simulink model "d_kundur2"  (Simulink 5.1)
settings: Solver=ode45  StartTime=0.0  StopTime=10.0  RelTol=1e-3
libraries: fm_lib x20
settings Model: Creator=fmilano  LastModifiedBy=fmilano  ExtModeAutoUpdateStatusClock=off  SignalLoggingName=logsout  BooleanDataType=on  RTWOptions="-aEnforceIntegerDowncast=1 -aFoldNonRolledExpr=1 -aInlineInvariantSignals=1 -aInlineParameters=0 -aLocalBlockOutputs=1 -aRollThreshold=5 -aZeroInternalMemoryAtStartup=1 -aZeroExternalMemoryAtStartup=1 -aInitFltsAndDblsToZero=1 -aForceBlockIOInitOptimize=0 -aGenerateReport=0 -aGenCodeOnly=0 -aRTWVerbose=1 -aIncludeHyperlinkInReport=0 -aLaunchReport=0 -aGenerateTraceInfo=0  -aForceParamTrailComments=0 -aGenerateComments=1 -aIgnoreCustomStorageClasses=1 -aIncHierarchyInIds=0 -aMaxRTWIdLen=31 -aShowEliminatedStatements=0 -aIncDataTypeInIds=0 -aInsertBlockDesc=0 -aIgnoreTestpoints=0 -aSimulinkBlockComments=1 -aInlinedPrmAccess=\"Literals\"  -aSuppressErrorStatus=0 -aModelReferenceCompliant=1 -aParenthesesLevel=\"Nominal\" -aModelStepFunctionPrototypeControlCompliant=0 -aPortableWordSizes=0 -aParMdlRefBuildCompliant=1 -aSupportNonInlinedSFcns=1 -aSupportContinuousTime=1 -aSupportComplex=1 -aSupportNonFinite=1 -aSupportAbsoluteTime=1 -aMultiwordLength=2048 -aTargetPreCompLibLocation=\"\" -aTargetLibSuffix=\"\" -aTargetFunctionLibrary=\"ANSI_C\" -aTargetFcnLib=\"ansi_tfl_tmw.mat\" -aMultiInstanceERTCode=0 -aLogVarNameModifier=\"rt_\" -aERTFirstTimeCompliant=0 -aIsPILTarget=0 -aCombineOutputUpdateFcns=0 -aGenerateASAP2=0 -aGenerateClassInterface=0 -aGenerateTestInterfaces=0 -aGenerateSampleERTMain=0 -aGenerateFullHeader=1 -aUtilityFuncGeneration=\"Auto\" -aIncludeFileDelimiter=\"Auto\" -aIncludeMdlTerminateFcn=1 -aPurelyIntegerCode=0 -aAutosarCompliant=0 -aERTCustomFileBanners=0 -aRTWCAPIStates=0 -aRTWCAPIParams=0 -aRTWCAPISignals=0 -aMatFileLogging=1 -aCompOptLevelCompliant=0 -aCPPClassGenCompliant=0 -aExtModeIntrfLevel=\"Level1\" -aExtModeMexFile=\"ext_comm\" -aExtModeTransport=0 -aExtModeStaticAllocSize=1000000 -aExtModeTesting=0 -aExtModeStaticAlloc=0 -aExtMode=0 -aERTMultiwordLength=256 -aERTMultiwordTypeDef=\"System defined\"  -aGenerateTraceInfo=0 -aGenerateTraceInfo=0 -aGenerateTraceInfo=0 -aGenerateTraceInfo=0"

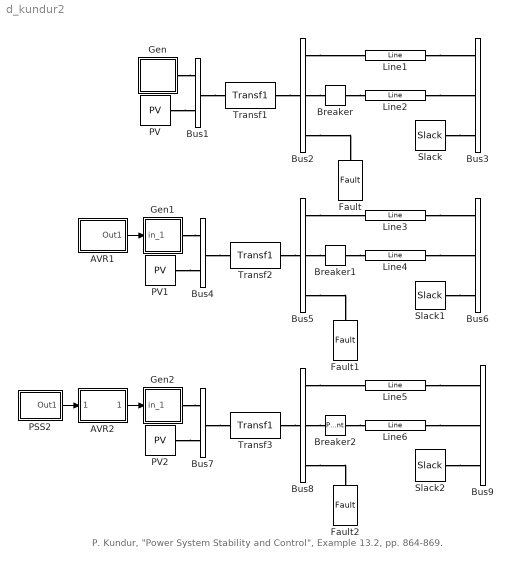
== system d_kundur2 ==
  note: P. Kundur, "Power System Stability and Control", Example 13.2, pp. 864-869.
  AVR1 : Subsystem  Tag=PSATblock  Description=Controls  mask(Exc){p2q=3, p3q=7.00, p4q=-6.40, p5q=200, p6q=1, p7q=1, p8q=1.00, p9q=0, p10q=0.0001, p11q=0.015, p12_13q=[0.0006  0.9], in=0}
      mask prompts: p2q "Automatic Voltage Regulator Type"; p3q "Maximum Regulator Voltage [p.u.]"; p4q "Minimum Regulator Voltage [p.u.]"; p5q "Regulator Gain [p.u./p.u.]"; p6q "Regulator Pole T2 [s]"; p7q "Regulator Zero T1 [s]"; p8q "Second Regulator Pole T3 [s]"; p9q "Allow signal V/V0 [0 for disabling signal]"; p10q "Time Constant of the Field Circuit Td [s]"; p11q "Time Delay of the Measurement System Tr [s]"; p12_13q "Coefficient of the Ceiling Function (A B)"; in "Number of input signals"
      mask help: This block defines an Automatic Voltage Regulator.
      mask init:
      | fm_inout
      | [x,y] = fm_draw('R');
      mask Help:
      | This block defines an Automatic Voltage Regulator.
      | There are three kind of regulators:
      | 
      | Type 1:
      | 
      |      IEEE Model 1
      | 
      | Type 2:
      | 
      |      IEEE Model 2
      | 
      | Type 3:
      | 
      |      IEEE Model 3
      mask StyleString: popup(1|2|3),edit,edit,edit,edit,edit,edit,edit,edit,edit,edit,popup(0|1|2|3)
      mask CallbackString: fm_block|||||||||||
      mask Display:
      | plot([-1.8 4.1 4.1 -1.8 -1.8],[-1.5 -1.5 1.5 1.5 -1.5])
      | color('red')
      | plot([-1.3 -0.5],[-1 1],[-0.5 0.3],[1 -1],[-0.9 -0.1],[0.0 0.0])
      | plot(2.8+1.3*x,2*y,1.5+[-1.3 -0.5],[1 -1],1.5+[-0.5 0.3],[-1 1])
  AVR2 : Subsystem  Tag=PSATblock  Description=Controls  mask(Exc){p2q=3, p3q=7.00, p4q=-6.40, p5q=200, p6q=1, p7q=1, p8q=1.00, p9q=0, p10q=0.0001, p11q=0.015, p12_13q=[0.0006  0.9], in=1}
      mask prompts: p2q "Automatic Voltage Regulator Type"; p3q "Maximum Regulator Voltage [p.u.]"; p4q "Minimum Regulator Voltage [p.u.]"; p5q "Regulator Gain [p.u./p.u.]"; p6q "Regulator Pole T2 [s]"; p7q "Regulator Zero T1 [s]"; p8q "Second Regulator Pole T3 [s]"; p9q "Allow signal V/V0 [0 for disabling signal]"; p10q "Time Constant of the Field Circuit Td [s]"; p11q "Time Delay of the Measurement System Tr [s]"; p12_13q "Coefficient of the Ceiling Function (A B)"; in "Number of input signals"
      mask help: This block defines an Automatic Voltage Regulator.
      mask init:
      | fm_inout
      | [x,y] = fm_draw('R');
      mask Help:
      | This block defines an Automatic Voltage Regulator.
      | There are three kind of regulators:
      | 
      | Type 1:
      | 
      |      IEEE Model 1
      | 
      | Type 2:
      | 
      |      IEEE Model 2
      | 
      | Type 3:
      | 
      |      IEEE Model 3
      mask StyleString: popup(1|2|3),edit,edit,edit,edit,edit,edit,edit,edit,edit,edit,popup(0|1|2|3)
      mask CallbackString: fm_block|||||||||||
      mask Display:
      | plot([-1.8 4.1 4.1 -1.8 -1.8],[-1.5 -1.5 1.5 1.5 -1.5])
      | color('red')
      | plot([-1.3 -0.5],[-1 1],[-0.5 0.3],[1 -1],[-0.9 -0.1],[0.0 0.0])
      | plot(2.8+1.3*x,2*y,1.5+[-1.3 -0.5],[1 -1],1.5+[-0.5 0.3],[-1 1])
  Breaker : fm_lib/Faults &  Breakers/Breaker  Tag=PSATblock  Description=Faults & Breakers  PhysicalDomain=psatdomain  SubClassName=unknown  LeftPortType=p1  RightPortType=p1  LConnTagsString=__newl0  RConnTagsString=__newr0  p3_4_5q="[2220  400  60]"  p6q=on  p7q=0.57  p8q=100  p9q=on  p10q=on
  Breaker1 : fm_lib/Faults &  Breakers/Breaker  Tag=PSATblock  Description=Faults & Breakers  PhysicalDomain=psatdomain  SubClassName=unknown  LeftPortType=p1  RightPortType=p1  LConnTagsString=__newl0  RConnTagsString=__newr0  p3_4_5q="[2220  400  60]"  p6q=on  p7q=0.57  p8q=100  p9q=on  p10q=on
  Breaker2 : PMComponent  Tag=PSATblock  Description=Faults & Breakers  PhysicalDomain=psatdomain  LeftPortType=p1  RightPortType=p1  LConnTagsString=__newl0  RConnTagsString=__newr0  mask(Breaker){p3_4_5q=[2220  400  60], p6q=on, p7q=0.57, p8q=100}
      mask prompts: p3_4_5q "Power, Voltage and Frequency Ratings [MVA, kV, Hz]"; p6q "Initially close"; p7q "First intervention time [s]"; p8q "Second intervention time [s]"
      mask help: This block defines a breaker.
      mask CallbackString: |fm_block||
      mask Display: plot([1 2 2 1 1],[-1 -1 1 1 -1]),color('red'),plot([1 2],[-1 1],[2 1],[-1 1])
  Bus1 : PMComponent  Tag=PSATblock  Description=Connection  PhysicalDomain=psatdomain  LeftPortType=p1  RightPortType=p1  LConnTagsString=__newl0|__newl1  RConnTagsString=__newr0  mask(Bus){in=2, out=1, p2q=400, p3_4q=[1.00   0.00], p5q=1, p6q=1}
      mask prompts: in "Number of inputs:"; out "Number of outputs:"; p2q "Voltage Rating [kV]"; p3_4q "Voltage initial guess [p.u.  rad]"; p5q "Area number"; p6q "Region number"
      mask help: Bus block.
      mask init:
      | fm_inout
      mask CallbackString: ||||fm_block|
      mask Display: plot([0 1 1 0 0],[0 0 1 1 0])
  Bus2 : PMComponent  Tag=PSATblock  Description=Connection  PhysicalDomain=psatdomain  LeftPortType=p1  RightPortType=p1  LConnTagsString=__newl0  RConnTagsString=__newr0|__newr1|__newr2  mask(Bus){in=1, out=3, p2q=400, p3_4q=[1.00   0.00], p5q=1, p6q=1}
      mask prompts: in "Number of inputs:"; out "Number of outputs:"; p2q "Voltage Rating [kV]"; p3_4q "Voltage initial guess [p.u.  rad]"; p5q "Area number"; p6q "Region number"
      mask help: Bus block.
      mask init:
      | fm_inout
      mask CallbackString: ||||fm_block|
      mask Display: plot([0 1 1 0 0],[0 0 1 1 0])
  Bus3 : PMComponent  Tag=PSATblock  Description=Connection  PhysicalDomain=psatdomain  LeftPortType=p1  RightPortType=p1  LConnTagsString=__newl0|__newl1|__newl2  mask(Bus){in=3, out=0, p2q=400, p3_4q=[1.00   0.00], p5q=1, p6q=1}
      mask prompts: in "Number of inputs:"; out "Number of outputs:"; p2q "Voltage Rating [kV]"; p3_4q "Voltage initial guess [p.u.  rad]"; p5q "Area number"; p6q "Region number"
      mask help: Bus block.
      mask init:
      | fm_inout
      mask CallbackString: ||||fm_block|
      mask Display: plot([0 1 1 0 0],[0 0 1 1 0])
  Bus4 : PMComponent  Tag=PSATblock  Description=Connection  PhysicalDomain=psatdomain  LeftPortType=p1  RightPortType=p1  LConnTagsString=__newl0|__newl1  RConnTagsString=__newr0  mask(Bus){in=2, out=1, p2q=400, p3_4q=[1.00   0.00], p5q=1, p6q=1}
      mask prompts: in "Number of inputs:"; out "Number of outputs:"; p2q "Voltage Rating [kV]"; p3_4q "Voltage initial guess [p.u.  rad]"; p5q "Area number"; p6q "Region number"
      mask help: Bus block.
      mask init:
      | fm_inout
      mask CallbackString: ||||fm_block|
      mask Display: plot([0 1 1 0 0],[0 0 1 1 0])
  Bus5 : PMComponent  Tag=PSATblock  Description=Connection  PhysicalDomain=psatdomain  LeftPortType=p1  RightPortType=p1  LConnTagsString=__newl0  RConnTagsString=__newr0|__newr1|__newr2  mask(Bus){in=1, out=3, p2q=400, p3_4q=[1.00   0.00], p5q=1, p6q=1}
      mask prompts: in "Number of inputs:"; out "Number of outputs:"; p2q "Voltage Rating [kV]"; p3_4q "Voltage initial guess [p.u.  rad]"; p5q "Area number"; p6q "Region number"
      mask help: Bus block.
      mask init:
      | fm_inout
      mask CallbackString: ||||fm_block|
      mask Display: plot([0 1 1 0 0],[0 0 1 1 0])
  Bus6 : PMComponent  Tag=PSATblock  Description=Connection  PhysicalDomain=psatdomain  LeftPortType=p1  RightPortType=p1  LConnTagsString=__newl0|__newl1|__newl2  mask(Bus){in=3, out=0, p2q=400, p3_4q=[1.00   0.00], p5q=1, p6q=1}
      mask prompts: in "Number of inputs:"; out "Number of outputs:"; p2q "Voltage Rating [kV]"; p3_4q "Voltage initial guess [p.u.  rad]"; p5q "Area number"; p6q "Region number"
      mask help: Bus block.
      mask init:
      | fm_inout
      mask CallbackString: ||||fm_block|
      mask Display: plot([0 1 1 0 0],[0 0 1 1 0])
  Bus7 : PMComponent  Tag=PSATblock  Description=Connection  PhysicalDomain=psatdomain  LeftPortType=p1  RightPortType=p1  LConnTagsString=__newl0|__newl1  RConnTagsString=__newr0  mask(Bus){in=2, out=1, p2q=400, p3_4q=[1.00   0.00], p5q=1, p6q=1}
      mask prompts: in "Number of inputs:"; out "Number of outputs:"; p2q "Voltage Rating [kV]"; p3_4q "Voltage initial guess [p.u.  rad]"; p5q "Area number"; p6q "Region number"
      mask help: Bus block.
      mask init:
      | fm_inout
      mask CallbackString: ||||fm_block|
      mask Display: plot([0 1 1 0 0],[0 0 1 1 0])
  Bus8 : PMComponent  Tag=PSATblock  Description=Connection  PhysicalDomain=psatdomain  LeftPortType=p1  RightPortType=p1  LConnTagsString=__newl0  RConnTagsString=__newr0|__newr1|__newr2  mask(Bus){in=1, out=3, p2q=400, p3_4q=[1.00   0.00], p5q=1, p6q=1}
      mask prompts: in "Number of inputs:"; out "Number of outputs:"; p2q "Voltage Rating [kV]"; p3_4q "Voltage initial guess [p.u.  rad]"; p5q "Area number"; p6q "Region number"
      mask help: Bus block.
      mask init:
      | fm_inout
      mask CallbackString: ||||fm_block|
      mask Display: plot([0 1 1 0 0],[0 0 1 1 0])
  Bus9 : PMComponent  Tag=PSATblock  Description=Connection  PhysicalDomain=psatdomain  LeftPortType=p1  RightPortType=p1  LConnTagsString=__newl0|__newl1|__newl2  mask(Bus){in=3, out=0, p2q=400, p3_4q=[1.00   0.00], p5q=1, p6q=1}
      mask prompts: in "Number of inputs:"; out "Number of outputs:"; p2q "Voltage Rating [kV]"; p3_4q "Voltage initial guess [p.u.  rad]"; p5q "Area number"; p6q "Region number"
      mask help: Bus block.
      mask init:
      | fm_inout
      mask CallbackString: ||||fm_block|
      mask Display: plot([0 1 1 0 0],[0 0 1 1 0])
  Fault : fm_lib/Faults &  Breakers/Fault  Tag=PSATblock  Description=Faults & Breakers  Orientation=down  PhysicalDomain=psatdomain  SubClassName=unknown  LeftPortType=p1  RightPortType=p1  LConnTagsString=__newl0  p2_3_4q="[2220  400  60]"  p5q=0.5  p6q=0.57  p7q=0  p8q=1e-5
  Fault1 : fm_lib/Faults &  Breakers/Fault  Tag=PSATblock  Description=Faults & Breakers  Orientation=down  PhysicalDomain=psatdomain  SubClassName=unknown  LeftPortType=p1  RightPortType=p1  LConnTagsString=__newl0  p2_3_4q="[2220  400  60]"  p5q=0.5  p6q=0.57  p7q=0  p8q=1e-5
  Fault2 : fm_lib/Faults &  Breakers/Fault  Tag=PSATblock  Description=Faults & Breakers  Orientation=down  PhysicalDomain=psatdomain  SubClassName=unknown  LeftPortType=p1  RightPortType=p1  LConnTagsString=__newl0  p2_3_4q="[2220  400  60]"  p5q=0.5  p6q=0.57  p7q=0  p8q=1e-5
  Gen : Subsystem  Tag=PSATblock  Description=Machines  mask(Syn){p2_3_4q=[2220  400   60], p5q=6, p7_6q=[0.003  0.15], p8_9_10q=[1.81  0.30  0.23], p11_12q=[8.00  0.03], p13_14_15q=[1.76  0.65  0.25], p16_17q=[1.00  0.07], p18_19q=[7.00  0.00], p20_21q=[0.00  0.00], p22_23q=[1.00  1.00], p24q=0.00, p25_26q=[0.05 0.1], in=0, p27q=0, p28q=on}
      mask prompts: p2_3_4q "Power, voltage and frequency ratings [MVA, kV, Hz]"; p5q "Machine Dynamic Order"; p7_6q "resistance ra and leakage reactance xl [p.u. p.u.]"; p8_9_10q "d-axis reactances Xd, X'd X"d [p.u.,p.u.,p.u.]"; p11_12q "d-axis open circuit time constants T'd0 and T"d0 [s, s]"; p13_14_15q "q-axis reactances Xq, X'q, X"q [p.u.  p.u.  p.u.]"; p16_17q "q-axis open circuit time constants T'q0 and T"q0 [s s]"; p18_19q "Inertia (M = 2H) and Damping [s, p.u.]"; p20_21q "Speed and active power additional signals Kw and Kp [p.u., p.u.]"; p22_23q "Percentage of active and reactive powers at bus [p.u. p.u.]"; p24q "d-axis additional circuit leakage time constant Taa [s]"; p25_26q "Saturation coefficients S(1.0) and S(1.2)"; in "Number of input signals"; p27q "COI number"; p28q "Connected"
      mask help: This block defines a fourth order synchronous machine.
      mask init:
      | fm_inout
      | [x,y] = fm_draw('circle');
      | [xg,yg] = fm_draw('G');
      | [xs,ys] = fm_draw('sinus');
      mask StyleString: edit,popup(8|6|5.3|5.2|5.1|4|3|2),edit,edit,edit,edit,edit,edit,edit,edit,edit,edit,popup(0|1|2),edit,checkbox
      mask CallbackString: |fm_block|||||||||||||fm_block
      mask Display:
      | plot(x+1.4,y,0.12*xs+1,0.15*ys-0.6)
      | color('blue')
      | plot(1.4+0.45*xg,0.3+0.45*yg)
  Gen1 : Subsystem  Tag=PSATblock  Description=Machines  mask(Syn){p2_3_4q=[2220  400   60], p5q=6, p7_6q=[0.003  0.15], p8_9_10q=[1.81  0.30  0.23], p11_12q=[8.00  0.03], p13_14_15q=[1.76  0.65  0.25], p16_17q=[1.00  0.07], p18_19q=[7.00  0.00], p20_21q=[0.00  0.00], p22_23q=[1.00  1.00], p24q=0.00, p25_26q=[0.05 0.1], in=1, p27q=0, p28q=on}
      mask prompts: p2_3_4q "Power, voltage and frequency ratings [MVA, kV, Hz]"; p5q "Machine Dynamic Order"; p7_6q "resistance ra and leakage reactance xl [p.u. p.u.]"; p8_9_10q "d-axis reactances Xd, X'd X"d [p.u.,p.u.,p.u.]"; p11_12q "d-axis open circuit time constants T'd0 and T"d0 [s, s]"; p13_14_15q "q-axis reactances Xq, X'q, X"q [p.u.  p.u.  p.u.]"; p16_17q "q-axis open circuit time constants T'q0 and T"q0 [s s]"; p18_19q "Inertia (M = 2H) and Damping [s, p.u.]"; p20_21q "Speed and active power additional signals Kw and Kp [p.u., p.u.]"; p22_23q "Percentage of active and reactive powers at bus [p.u. p.u.]"; p24q "d-axis additional circuit leakage time constant Taa [s]"; p25_26q "Saturation coefficients S(1.0) and S(1.2)"; in "Number of input signals"; p27q "COI number"; p28q "Connected"
      mask help: This block defines a fourth order synchronous machine.
      mask init:
      | fm_inout
      | [x,y] = fm_draw('circle');
      | [xg,yg] = fm_draw('G');
      | [xs,ys] = fm_draw('sinus');
      mask StyleString: edit,popup(8|6|5.3|5.2|5.1|4|3|2),edit,edit,edit,edit,edit,edit,edit,edit,edit,edit,popup(0|1|2),edit,checkbox
      mask CallbackString: |fm_block|||||||||||||fm_block
      mask Display:
      | plot(x+1.4,y,0.12*xs+1,0.15*ys-0.6)
      | color('blue')
      | plot(1.4+0.45*xg,0.3+0.45*yg)
  Gen2 : Subsystem  Tag=PSATblock  Description=Machines  mask(Syn){p2_3_4q=[2220  400   60], p5q=6, p7_6q=[0.003  0.15], p8_9_10q=[1.81  0.30  0.23], p11_12q=[8.00  0.03], p13_14_15q=[1.76  0.65  0.25], p16_17q=[1.00  0.07], p18_19q=[7.00  0.00], p20_21q=[0.00  0.00], p22_23q=[1.00  1.00], p24q=0.00, p25_26q=[0.05  0.1], in=1, p27q=0, p28q=on}
      mask prompts: p2_3_4q "Power, voltage and frequency ratings [MVA, kV, Hz]"; p5q "Machine Dynamic Order"; p7_6q "resistance ra and leakage reactance xl [p.u. p.u.]"; p8_9_10q "d-axis reactances Xd, X'd X"d [p.u.,p.u.,p.u.]"; p11_12q "d-axis open circuit time constants T'd0 and T"d0 [s, s]"; p13_14_15q "q-axis reactances Xq, X'q, X"q [p.u.  p.u.  p.u.]"; p16_17q "q-axis open circuit time constants T'q0 and T"q0 [s s]"; p18_19q "Inertia (M = 2H) and Damping [s, p.u.]"; p20_21q "Speed and active power additional signals Kw and Kp [p.u., p.u.]"; p22_23q "Percentage of active and reactive powers at bus [p.u. p.u.]"; p24q "d-axis additional circuit leakage time constant Taa [s]"; p25_26q "Saturation coefficients S(1.0) and S(1.2)"; in "Number of input signals"; p27q "COI number"; p28q "Connected"
      mask help: This block defines a fourth order synchronous machine.
      mask init:
      | fm_inout
      | [x,y] = fm_draw('circle');
      | [xg,yg] = fm_draw('G');
      | [xs,ys] = fm_draw('sinus');
      mask StyleString: edit,popup(8|6|5.3|5.2|5.1|4|3|2),edit,edit,edit,edit,edit,edit,edit,edit,edit,edit,popup(0|1|2),edit,checkbox
      mask CallbackString: |fm_block|||||||||||||fm_block
      mask Display:
      | plot(x+1.4,y,0.12*xs+1,0.15*ys-0.6)
      | color('blue')
      | plot(1.4+0.45*xg,0.3+0.45*yg)
  Line1 : fm_lib/Power Flow/Line  Tag=PSATblock  Description=Power Flow  PhysicalDomain=psatdomain  SubClassName=unknown  LeftPortType=p1  RightPortType=p1  LConnTagsString=__newl0  RConnTagsString=__newr0  p3_4_5q="[2220  400  60]"  p6q=0  p8q=0.0  p9q=0.5  p10q=0.0  p13_14_15q="[0.0  0.0  0.0]"  p16q=on
  Line2 : fm_lib/Power Flow/Line  Tag=PSATblock  Description=Power Flow  PhysicalDomain=psatdomain  SubClassName=unknown  LeftPortType=p1  RightPortType=p1  LConnTagsString=__newl0  RConnTagsString=__newr0  p3_4_5q="[2220  400  60]"  p6q=0  p8q=0.0  p9q=0.93  p10q=0.0  p13_14_15q="[0.0  0.0  0.0]"  p16q=on
  Line3 : fm_lib/Power Flow/Line  Tag=PSATblock  Description=Power Flow  PhysicalDomain=psatdomain  SubClassName=unknown  LeftPortType=p1  RightPortType=p1  LConnTagsString=__newl0  RConnTagsString=__newr0  p3_4_5q="[2220  400  60]"  p6q=0  p8q=0.0  p9q=0.5  p10q=0.0  p13_14_15q="[0.0  0.0  0.0]"  p16q=on
  Line4 : fm_lib/Power Flow/Line  Tag=PSATblock  Description=Power Flow  PhysicalDomain=psatdomain  SubClassName=unknown  LeftPortType=p1  RightPortType=p1  LConnTagsString=__newl0  RConnTagsString=__newr0  p3_4_5q="[2220  400  60]"  p6q=0  p8q=0.0  p9q=0.93  p10q=0.0  p13_14_15q="[0.0  0.0  0.0]"  p16q=on
  Line5 : fm_lib/Power Flow/Line  Tag=PSATblock  Description=Power Flow  PhysicalDomain=psatdomain  SubClassName=unknown  LeftPortType=p1  RightPortType=p1  LConnTagsString=__newl0  RConnTagsString=__newr0  p3_4_5q="[2220  400  60]"  p6q=0  p8q=0.0  p9q=0.5  p10q=0.0  p13_14_15q="[0.0  0.0  0.0]"  p16q=on
  Line6 : fm_lib/Power Flow/Line  Tag=PSATblock  Description=Power Flow  PhysicalDomain=psatdomain  SubClassName=unknown  LeftPortType=p1  RightPortType=p1  LConnTagsString=__newl0  RConnTagsString=__newr0  p3_4_5q="[2220  400  60]"  p6q=0  p8q=0.0  p9q=0.93  p10q=0.0  p13_14_15q="[0.0  0.0  0.0]"  p16q=on
  PSS2 : Subsystem  Tag=PSATblock  Description=Controls  mask(Pss){p2q=2, p3q=omega, p4_5q=[0.2 -0.2], p6_7q=[9.5  1.41], p14_15q=20  5, p8_9_10_11q=[0.154 0.033 1 1], p12_13q=[25 0.5], p16_17_18_19q=[0.045  0.045  0.045  -0.045], p20_21q=[1.000  0.95], p22q=off, p23q=on}
      mask prompts: p2q "PSS model"; p3q "Input Signal"; p4_5q "Max and Min Stabilizer Output [p.u.]"; p6_7q "Gain Kw and time constant Tw  [p.u./p.u., s]"; p14_15q "Electrical power gain Kp and voltage gain Kv [p.u./p.u., p.u./p.u.]"; p8_9_10_11q "Lead-Lag time constants T1, T2, T3, T4 [s, s, s, s]"; p12_13q "Gain Ka and time constant Ta [p.u./p.u., s]"; p16_17_18_19q "Additional signal limits Va_max, Va_thr, V3_max and V3_min [p.u., p.u., p.u., p.u.]"; p20_21q "Threshold limits E_thr and w_thr [p.u., p.u.]"; p22q "Allow switch S2"; p23q "Connected"
      mask help: This block defines a Power System Stabilizer.
      mask init:
      | [xs,ys] = fm_draw('S');
      | [xp,yp] = fm_draw('P');
      mask StyleString: popup(1|2|3|4|5),popup(omega|power|voltage),edit,edit,edit,edit,edit,edit,edit,checkbox,checkbox
      mask CallbackString: fm_block||||||||||fm_block
      mask Display:
      | plot([-1.8 4.1 4.1 -1.8 -1.8],[-1.5 -1.5 1.5 1.5 -1.5])
      | color('red')
      | plot(1.5*xp-0.7,2*yp,1.2+1.5*xs,2*ys,2.8+1.5*xs,2*ys)
  PV : fm_lib/Power Flow/PV  Tag=PSATblock  Description=Power Flow  PhysicalDomain=psatdomain  SubClassName=unknown  LeftPortType=p1  RightPortType=p1  RConnTagsString=__newr0  p2_3q="[2220  400]"  p4q=0.9  p5q=1.00  p6_7q="[0.8  -0.2]"  p8_9q="[1.1  0.9]"  p10q=1  p11q=on
  PV1 : fm_lib/Power Flow/PV  Tag=PSATblock  Description=Power Flow  PhysicalDomain=psatdomain  SubClassName=unknown  LeftPortType=p1  RightPortType=p1  RConnTagsString=__newr0  p2_3q="[2220  400]"  p4q=0.9  p5q=1.00  p6_7q="[0.8  -0.2]"  p8_9q="[1.1  0.9]"  p10q=1  p11q=on
  PV2 : fm_lib/Power Flow/PV  Tag=PSATblock  Description=Power Flow  PhysicalDomain=psatdomain  SubClassName=unknown  LeftPortType=p1  RightPortType=p1  RConnTagsString=__newr0  p2_3q="[2220  400]"  p4q=0.9  p5q=1.00  p6_7q="[0.8  -0.2]"  p8_9q="[1.1  0.9]"  p10q=1  p11q=on
  Slack : fm_lib/Power Flow/Slack  Tag=PSATblock  Description=Power Flow  PhysicalDomain=psatdomain  SubClassName=unknown  LeftPortType=p1  RightPortType=p1  RConnTagsString=__newr0  p2_3q="[2220  400]"  p4q=0.90081  p5q=0.00  p6_7q="[1.5  -1.5]"  p8_9q="[1.1  0.9]"  p10q=0.80  p11q=1  p12q=on  p13q=on
  Slack1 : fm_lib/Power Flow/Slack  Tag=PSATblock  Description=Power Flow  PhysicalDomain=psatdomain  SubClassName=unknown  LeftPortType=p1  RightPortType=p1  RConnTagsString=__newr0  p2_3q="[2220  400]"  p4q=0.90081  p5q=0.00  p6_7q="[1.5  -1.5]"  p8_9q="[1.1  0.9]"  p10q=0.80  p11q=1  p12q=on  p13q=on
  Slack2 : fm_lib/Power Flow/Slack  Tag=PSATblock  Description=Power Flow  PhysicalDomain=psatdomain  SubClassName=unknown  LeftPortType=p1  RightPortType=p1  RConnTagsString=__newr0  p2_3q="[2220  400]"  p4q=0.90081  p5q=0.00  p6_7q="[1.5  -1.5]"  p8_9q="[1.1  0.9]"  p10q=0.80  p11q=1  p12q=on  p13q=on
  Transf1 : fm_lib/Power Flow/Transf1  Tag=PSATblock  Description=Power Flow  PhysicalDomain=psatdomain  SubClassName=unknown  LeftPortType=p1  RightPortType=p1  LConnTagsString=__newl0  RConnTagsString=__newr0  p3_4_5q="[2220  400  60]"  p7q=1  p8q=0.0  p9q=0.15  p13_14_15q="[0.0  0.0  0.0]"  p16q=on
  Transf2 : fm_lib/Power Flow/Transf1  Tag=PSATblock  Description=Power Flow  PhysicalDomain=psatdomain  SubClassName=unknown  LeftPortType=p1  RightPortType=p1  LConnTagsString=__newl0  RConnTagsString=__newr0  p3_4_5q="[2220  400  60]"  p7q=1  p8q=0.0  p9q=0.15  p13_14_15q="[0.0  0.0  0.0]"  p16q=on
  Transf3 : fm_lib/Power Flow/Transf1  Tag=PSATblock  Description=Power Flow  PhysicalDomain=psatdomain  SubClassName=unknown  LeftPortType=p1  RightPortType=p1  LConnTagsString=__newl0  RConnTagsString=__newr0  p3_4_5q="[2220  400  60]"  p7q=1  p8q=0.0  p9q=0.15  p13_14_15q="[0.0  0.0  0.0]"  p16q=on
  wires:
  PSS2/1(Out1) -> AVR2/1(in_1)
  AVR2/1(Out1) -> Gen2/1(in_1)
  AVR1/1(Out1) -> Gen1/1(in_1)
  connections:
  Bus8/RConn3 -- Fault2/LConn1
  Breaker2/RConn1 -- Line6/LConn1
  Slack2/RConn1 -- Bus9/LConn3
  Line6/RConn1 -- Bus9/LConn2
  Line5/RConn1 -- Bus9/LConn1
  Bus8/RConn1 -- Line5/LConn1
  Bus8/RConn2 -- Breaker2/LConn1
  Transf3/RConn1 -- Bus8/LConn1
  Bus7/RConn1 -- Transf3/LConn1
  PV2/RConn1 -- Bus7/LConn2
  Gen2/RConn1 -- Bus7/LConn1
  Bus5/RConn3 -- Fault1/LConn1
  Breaker1/RConn1 -- Line4/LConn1
  Slack1/RConn1 -- Bus6/LConn3
  Line4/RConn1 -- Bus6/LConn2
  Line3/RConn1 -- Bus6/LConn1
  Bus5/RConn1 -- Line3/LConn1
  Bus5/RConn2 -- Breaker1/LConn1
  Transf2/RConn1 -- Bus5/LConn1
  Bus4/RConn1 -- Transf2/LConn1
  PV1/RConn1 -- Bus4/LConn2
  Gen1/RConn1 -- Bus4/LConn1
  Bus2/RConn3 -- Fault/LConn1
  Breaker/RConn1 -- Line2/LConn1
  Slack/RConn1 -- Bus3/LConn3
  Line2/RConn1 -- Bus3/LConn2
  Line1/RConn1 -- Bus3/LConn1
  Bus2/RConn1 -- Line1/LConn1
  Bus2/RConn2 -- Breaker/LConn1
  Transf1/RConn1 -- Bus2/LConn1
  Bus1/RConn1 -- Transf1/LConn1
  PV/RConn1 -- Bus1/LConn2
  Gen/RConn1 -- Bus1/LConn1

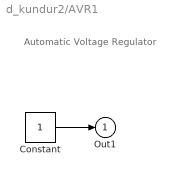
== system d_kundur2/AVR1 ==
  note: Automatic Voltage Regulator
  Constant : Constant  OutDataType=sfix(16)  OutScaling=2^0
  Out1 : Outport
  wires:
  Constant/1 -> Out1/1

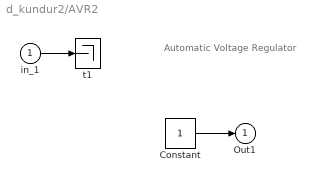
== system d_kundur2/AVR2 ==
  note: Automatic Voltage Regulator
  in_1 : Inport  OutDataType=sfix(16)  OutScaling=2^0
  Constant : Constant  OutDataType=sfix(16)  OutScaling=2^0
  t1 : Terminator
  Out1 : Outport
  wires:
  in_1/1 -> t1/1
  Constant/1 -> Out1/1

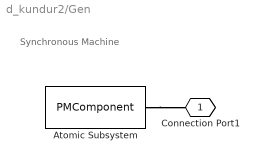
== system d_kundur2/Gen ==
  note: Synchronous Machine
  Atomic Subsystem : PMComponent  PhysicalDomain=psatdomain  LeftPortType=p1  RightPortType=p1  RConnTagsString=__newr0
  Connection Port1 : PMIOPort  Tag=PMCPort  Orientation=left  Port=1  Side=Right
  connections:
  Atomic Subsystem/RConn1 -- Connection Port1/RConn1

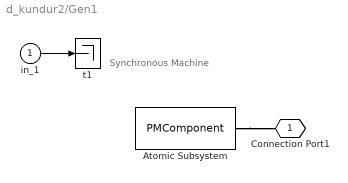
== system d_kundur2/Gen1 ==
  note: Synchronous Machine
  in_1 : Inport
  Atomic Subsystem : PMComponent  PhysicalDomain=psatdomain  LeftPortType=p1  RightPortType=p1  RConnTagsString=__newr0
  t1 : Terminator
  Connection Port1 : PMIOPort  Tag=PMCPort  Orientation=left  Port=1  Side=Right
  wires:
  in_1/1 -> t1/1
  connections:
  Atomic Subsystem/RConn1 -- Connection Port1/RConn1

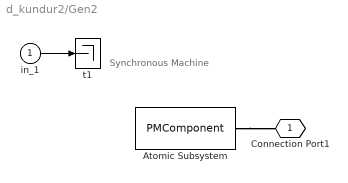
== system d_kundur2/Gen2 ==
  note: Synchronous Machine
  in_1 : Inport
  Atomic Subsystem : PMComponent  PhysicalDomain=psatdomain  LeftPortType=p1  RightPortType=p1  RConnTagsString=__newr0
  t1 : Terminator
  Connection Port1 : PMIOPort  Tag=PMCPort  Orientation=left  Port=1  Side=Right
  wires:
  in_1/1 -> t1/1
  connections:
  Atomic Subsystem/RConn1 -- Connection Port1/RConn1

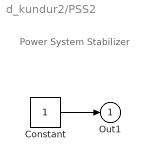
== system d_kundur2/PSS2 ==
  note: Power System Stabilizer
  Constant : Constant  OutDataType=sfix(16)  OutScaling=2^0
  Out1 : Outport
  wires:
  Constant/1 -> Out1/1
